simulink model "motor"  (R2017b)
settings: Solver=VariableStepAuto  StartTime=0.0  StopTime=1  RelTol=1e-3
values from neighbouring files (symbols this model uses):
  Amp1d = [1]    [System.m]
  Amp1n = [Vss]    [System.m]
  AmpSat1 = NomVoltage    [System.m]
  BackEMF1 = 1/KEmf    [System.m]
  Elec1d = [La Ra]    [System.m]
  Elec1n = [1]    [System.m]
  JntSat1 = JntLim * RadPerDeg    [System.m]
  Mech1d = [JRotor KineticFriction 0]    [System.m]
  Mech1n = [1 0]    [System.m]
  NomCurrent = 3.2    [CONSTANTS.m]
  PID1 = [1 0 2.6]    [System.m]
  StallCurrent = 6.031    [CONSTANTS.m]
  TConst1 = KTorque    [System.m]
libraries: simulink x5
settings Model: Creator=Moochster  LastModifiedBy=lucyl

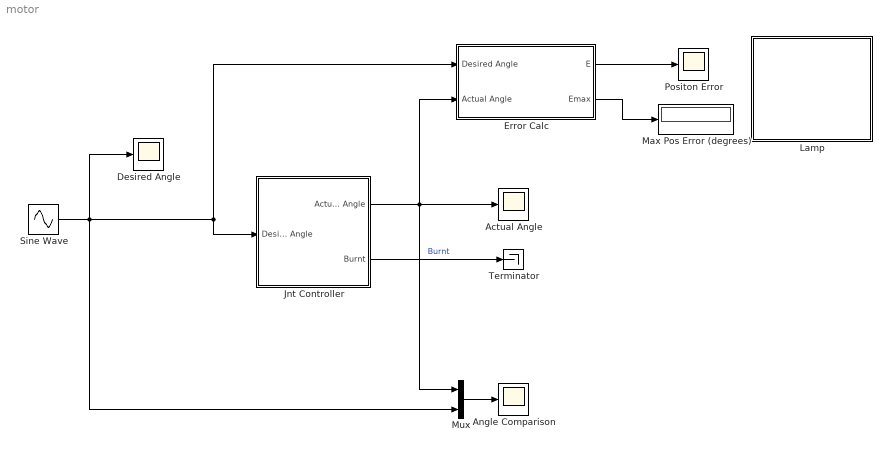
== system motor ==
  Actual Angle : Scope
  Angle Comparison : Scope
  Desired Angle : Scope
  Error Calc : Subsystem
  Jnt Controller : Subsystem
  Lamp : Subsystem  DialogController=hmiCreateDDGDialog  IsWebBlock=on  mask(MWDashboardBlock){webBlockId=7fcfd6b5-b98b-441a-9880-35fe4990fbef, webBlockType=lamp, ShowInLibBrowser=on, ShowInitialText=on, HMISrcModelName=motor}
      mask prompts: webBlockType "WebBlock Type"; HMISrcModelName "Source Model"
      mask help: SimulinkHMI:dialogs:LampDialogDesc
      mask Help: helpview([docroot '/mapfiles/simulink.map'], 'hmi_lamp')
      mask Display:
      | if strcmp(get_param(bdroot(gcb),'BlockDiagramType'), 'library')
      |     image([(matlabroot) '/toolbox/simulink/hmi/icons/Lamp.png']);
      | end
  Max Pos Error (degrees) : Display
  Mux : Mux  Inputs=2
  Positon Error : Scope
  Sine Wave : Sin  Amplitude=pi/4  Frequency=15*2*pi  Samples=15  SampleTime=0
  Terminator : Terminator
  wires:
  Sine Wave/1 -> Mux/2, Desired Angle/1, Error Calc/1(Desired Angle), Jnt Controller/1(Desired Angle)
  Jnt Controller/1(Actual Angle) -> Error Calc/2(Actual Angle), Actual Angle/1, Mux/1
  Error Calc/1(E) -> Positon Error/1
  Error Calc/2(Emax) -> Max Pos Error (degrees)/1
  Jnt Controller/2(Burnt) -> Terminator/1  "Burnt"
  Mux/1 -> Angle Comparison/1

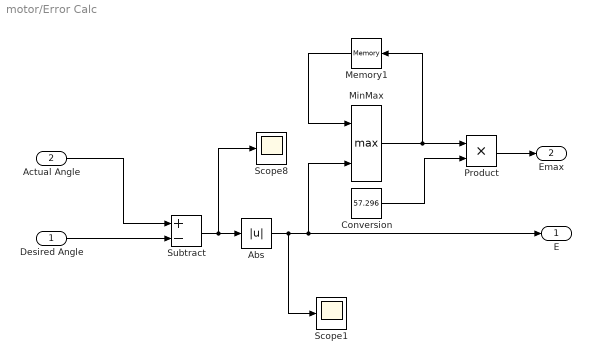
== system motor/Error Calc ==
  Desired Angle : Inport
  Actual Angle : Inport  Port=2
  Abs : Abs
  Conversion : Constant  Value=57.296
  Memory1 : Memory
  MinMax : MinMax  Function=max  Inputs=2  ZeroCross=off
  Product : Product
  Scope1 : Scope
  Scope8 : Scope
  Subtract : Sum  Inputs=+-
  E : Outport
  Emax : Outport  Port=2
  wires:
  Actual Angle/1 -> Subtract/1
  Desired Angle/1 -> Subtract/2
  Subtract/1 -> Scope8/1, Abs/1
  MinMax/1 -> Product/1, Memory1/1
  Memory1/1 -> MinMax/1
  Abs/1 -> Scope1/1, MinMax/2, E/1
  Product/1 -> Emax/1
  Conversion/1 -> Product/2

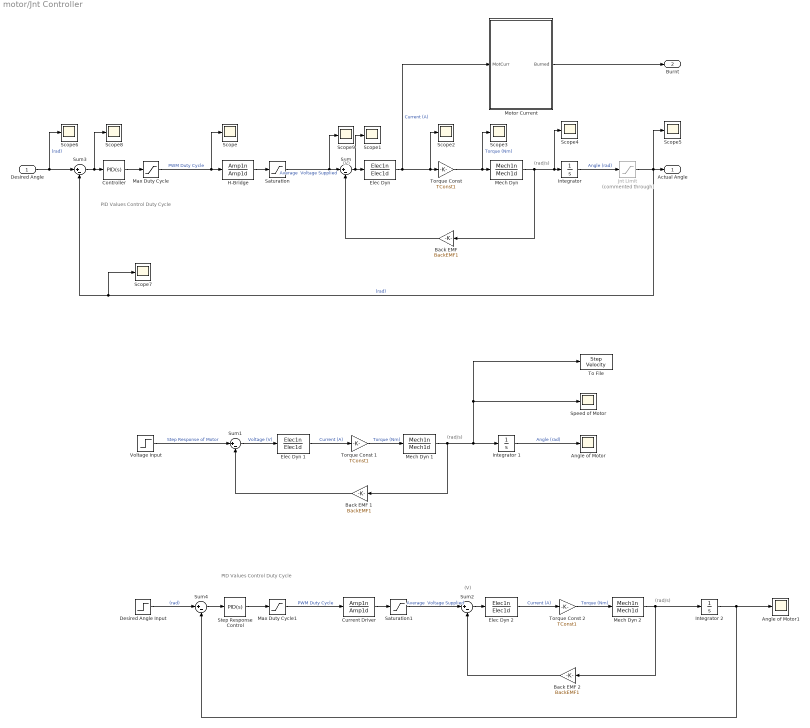
== system motor/Jnt Controller ==
  note: (rad/s)
  note: (V)
  note: PID Values Control Duty Cycle
  note: (rad/s)
  note: (rad/s)
  note: (V)
  note: PID Values Control Duty Cycle
  Desired Angle : Inport
  Angle of Motor : Scope
  Angle of Motor1 : Scope
  "Back EMF " : Gain  Gain=BackEMF1
  Back EMF 1 : Gain  Gain=BackEMF1
  Back EMF 2 : Gain  Gain=BackEMF1
  "Controller " : simulink/Continuous/PID Controller  Controller=PID  TimeDomain=Continuous-time  SampleTime=-1  IntegratorMethod=Forward Euler  FilterMethod=Forward Euler  Form=Parallel  UseFilter=on  ControllerParametersSource=internal  P=PID1(1)  I=PID1(2)  D=PID1(3)  N=100  InitialConditionSource=internal  InitialConditionForIntegrator=0  InitialConditionForFilter=0  ExternalReset=none  LimitOutput=off  UpperSaturationLimit=inf  LowerSaturationLimit=-inf  LinearizeAsGain=on  AntiWindupMode=none  Kb=1  TrackingMode=off  Kt=1  PParamMin=[]  PParamMax=[]  IParamMin=[]  IParamMax=[]  DParamMin=[]  DParamMax=[]  NParamMin=[]  NParamMax=[]  KbParamMin=[]  KbParamMax=[]  KtParamMin=[]  KtParamMax=[]  POutMin=[]  POutMax=[]  IOutMin=[]  IOutMax=[]  DOutMin=[]  DOutMax=[]  NOutMin=[]  NOutMax=[]  KbOutMin=[]  KbOutMax=[]  KtOutMin=[]  KtOutMax=[]  IntegratorOutMin=[]  IntegratorOutMax=[]  FilterOutMin=[]  FilterOutMax=[]  SumOutMin=[]  SumOutMax=[]  SumI1OutMin=[]  SumI1OutMax=[]  SumI2OutMin=[]  SumI2OutMax=[]  SumI3OutMin=[]  SumI3OutMax=[]  SumDOutMin=[]  SumDOutMax=[]  SaturationOutMin=[]  SaturationOutMax=[]  IntegratorContinuousStateAttributes=''  IntegratorStateMustResolveToSignalObject=off  IntegratorRTWStateStorageClass=Auto  FilterContinuousStateAttributes=''  FilterStateMustResolveToSignalObject=off  FilterRTWStateStorageClass=Auto  DifferentiatorICPrevScaledInput=0  DifferentiatorOutMin=[]  DifferentiatorOutMax=[]  InitialConditionSetting=State (most efficient)  FilterDiffOutCoefMin=[]  FilterDiffOutCoefMax=[]  SumDenOutMin=[]  SumDenOutMax=[]  SumNumOutMin=[]  SumNumOutMax=[]  ReciprocalOutMin=[]  ReciprocalOutMax=[]  DivideOutMin=[]  DivideOutMax=[]  TunerSelectOption=Transfer Function Based (PID Tuner App)
  Current Driver : TransferFcn  Numerator=Amp1n  Denominator=Amp1d
  Desired Angle Input : Step  Time=0  SampleTime=0
  "Elec Dyn " : TransferFcn  Numerator=Elec1n  Denominator=Elec1d
  Elec Dyn 1 : TransferFcn  Numerator=Elec1n  Denominator=Elec1d
  Elec Dyn 2 : TransferFcn  Numerator=Elec1n  Denominator=Elec1d
  "H-Bridge " : TransferFcn  Numerator=Amp1n  Denominator=Amp1d
  "Integrator " : Integrator
  Integrator 1 : Integrator
  Integrator 2 : Integrator
  "Jnt Limit " : Saturate  Commented=through  UpperLimit=JntSat1  LowerLimit=-JntSat1
  Max Duty Cycle : Saturate  UpperLimit=1  LowerLimit=-1
  Max Duty Cycle1 : Saturate  UpperLimit=1  LowerLimit=-1
  "Mech Dyn " : TransferFcn  Numerator=Mech1n  Denominator=Mech1d
  Mech Dyn 1 : TransferFcn  Numerator=Mech1n  Denominator=Mech1d
  Mech Dyn 2 : TransferFcn  Numerator=Mech1n  Denominator=Mech1d
  Motor Current : Subsystem
  Saturation : Saturate  UpperLimit=AmpSat1  LowerLimit=-AmpSat1
  Saturation1 : Saturate  UpperLimit=AmpSat1  LowerLimit=-AmpSat1
  Scope{,1..9} (10 alike) : Scope
  Speed of Motor : Scope
  Step Response Control : simulink/Continuous/PID Controller  Controller=PID  TimeDomain=Continuous-time  SampleTime=-1  IntegratorMethod=Forward Euler  FilterMethod=Forward Euler  Form=Parallel  UseFilter=on  ControllerParametersSource=internal  P=PID1(1)  I=PID1(2)  D=PID1(3)  N=100  InitialConditionSource=internal  InitialConditionForIntegrator=0  InitialConditionForFilter=0  ExternalReset=none  LimitOutput=off  UpperSaturationLimit=inf  LowerSaturationLimit=-inf  LinearizeAsGain=on  AntiWindupMode=none  Kb=1  TrackingMode=off  Kt=1  PParamMin=[]  PParamMax=[]  IParamMin=[]  IParamMax=[]  DParamMin=[]  DParamMax=[]  NParamMin=[]  NParamMax=[]  KbParamMin=[]  KbParamMax=[]  KtParamMin=[]  KtParamMax=[]  POutMin=[]  POutMax=[]  IOutMin=[]  IOutMax=[]  DOutMin=[]  DOutMax=[]  NOutMin=[]  NOutMax=[]  KbOutMin=[]  KbOutMax=[]  KtOutMin=[]  KtOutMax=[]  IntegratorOutMin=[]  IntegratorOutMax=[]  FilterOutMin=[]  FilterOutMax=[]  SumOutMin=[]  SumOutMax=[]  SumI1OutMin=[]  SumI1OutMax=[]  SumI2OutMin=[]  SumI2OutMax=[]  SumI3OutMin=[]  SumI3OutMax=[]  SumDOutMin=[]  SumDOutMax=[]  SaturationOutMin=[]  SaturationOutMax=[]  IntegratorContinuousStateAttributes=''  IntegratorStateMustResolveToSignalObject=off  IntegratorRTWStateStorageClass=Auto  FilterContinuousStateAttributes=''  FilterStateMustResolveToSignalObject=off  FilterRTWStateStorageClass=Auto  DifferentiatorICPrevScaledInput=0  DifferentiatorOutMin=[]  DifferentiatorOutMax=[]  InitialConditionSetting=State (most efficient)  FilterDiffOutCoefMin=[]  FilterDiffOutCoefMax=[]  SumDenOutMin=[]  SumDenOutMax=[]  SumNumOutMin=[]  SumNumOutMax=[]  ReciprocalOutMin=[]  ReciprocalOutMax=[]  DivideOutMin=[]  DivideOutMax=[]  TunerSelectOption=Transfer Function Based (PID Tuner App)
  Sum{,1..4} (5 alike) : Sum  Inputs=|+-
  To File : ToFile  Filename=Step Velocity  SampleTime=0.01
  "Torque Const " : Gain  Gain=TConst1
  Torque Const 1 : Gain  Gain=TConst1
  Torque Const 2 : Gain  Gain=TConst1
  Voltage Input : Step  Time=0.02  After=4.12  SampleTime=0
  Actual Angle : Outport
  Burnt : Outport  Port=2
  wires:
  "Controller "/1 -> Max Duty Cycle/1
  Sum/1 -> Scope1/1, "Elec Dyn "/1
  Sum3/1 -> Scope8/1, "Controller "/1
  "Elec Dyn "/1 -> Motor Current/1(MotCurr), Scope2/1, "Torque Const "/1  "Current (A)"
  "H-Bridge "/1 -> Saturation/1
  "Back EMF "/1 -> Sum/2
  "Jnt Limit "/1 -> Scope5/1, Actual Angle/1, Scope7/1, Sum3/2  "(rad)"
  Desired Angle/1 -> Scope6/1, Sum3/1  "(rad)"
  "Torque Const "/1 -> Scope3/1, "Mech Dyn "/1  "Torque (Nm)"
  "Integrator "/1 -> "Jnt Limit "/1  "Angle (rad)"
  "Mech Dyn "/1 -> Scope4/1, "Integrator "/1, "Back EMF "/1
  Saturation/1 -> Scope9/1, Sum/1  "Average  Voltage Supplied"
  Motor Current/1(Burned) -> Burnt/1
  Max Duty Cycle/1 -> Scope/1, "H-Bridge "/1  "PWM Duty Cycle"
  Mech Dyn 1/1 -> Back EMF 1/1, Integrator 1/1, To File/1, Speed of Motor/1
  Integrator 1/1 -> Angle of Motor/1  "Angle (rad)"
  Torque Const 1/1 -> Mech Dyn 1/1  "Torque (Nm)"
  Voltage Input/1 -> Sum1/1  "Step Response of Motor"
  Back EMF 1/1 -> Sum1/2
  Elec Dyn 1/1 -> Torque Const 1/1  "Current (A)"
  Sum1/1 -> Elec Dyn 1/1  "Voltage (V)"
  Max Duty Cycle1/1 -> Current Driver/1  "PWM Duty Cycle"
  Saturation1/1 -> Sum2/1  "Average  Voltage Supplied"
  Mech Dyn 2/1 -> Back EMF 2/1, Integrator 2/1
  Integrator 2/1 -> Angle of Motor1/1, Sum4/2
  Torque Const 2/1 -> Mech Dyn 2/1  "Torque (Nm)"
  Desired Angle Input/1 -> Sum4/1  "(rad)"
  Back EMF 2/1 -> Sum2/2
  Current Driver/1 -> Saturation1/1
  Elec Dyn 2/1 -> Torque Const 2/1  "Current (A)"
  Sum4/1 -> Step Response Control/1
  Sum2/1 -> Elec Dyn 2/1
  Step Response Control/1 -> Max Duty Cycle1/1

== system motor/Lamp ==

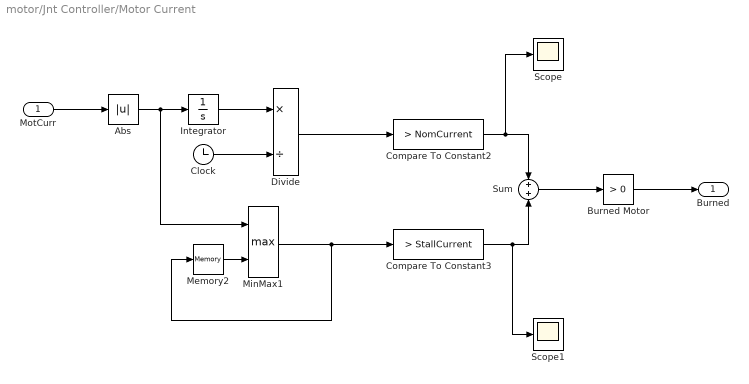
== system motor/Jnt Controller/Motor Current ==
  MotCurr : Inport
  Abs : Abs
  Burned Motor : simulink/Logic and Bit Operations/Compare To Zero  relop=>  OutDataTypeStr=boolean
  Clock : Clock
  Compare To Constant2 : simulink/Logic and Bit Operations/Compare To Constant  relop=>  const=NomCurrent  OutDataTypeStr=boolean
  Compare To Constant3 : simulink/Logic and Bit Operations/Compare To Constant  relop=>  const=StallCurrent  OutDataTypeStr=boolean
  Divide : Product  Inputs=*/
  Integrator : Integrator
  Memory2 : Memory
  MinMax1 : MinMax  Function=max  Inputs=2  ZeroCross=off
  Scope : Scope
  Scope1 : Scope
  Sum : Sum
  Burned : Outport
  wires:
  Sum/1 -> Burned Motor/1
  Burned Motor/1 -> Burned/1
  Memory2/1 -> MinMax1/2
  Compare To Constant2/1 -> Scope/1, Sum/1
  Compare To Constant3/1 -> Scope1/1, Sum/2
  MinMax1/1 -> Memory2/1, Compare To Constant3/1
  Divide/1 -> Compare To Constant2/1
  Abs/1 -> Integrator/1, MinMax1/1
  Clock/1 -> Divide/2
  Integrator/1 -> Divide/1
  MotCurr/1 -> Abs/1
